simulink model "satellite2"  (R2025b)
settings: Solver=FixedStepAuto  StartTime=0.0  StopTime=5000  FixedStep=dt  MinStep=0.0001  RelTol=1e-3
values from neighbouring files (symbols this model uses):
  A_mw = [ ... (first row only)    [init_params.m]
  A_w = [ ... (first row only)    [init_params.m]
  alpha1 = 0.1    [init_params.m]
  alpha2 = 0.1    [init_params.m]
  angle0 = eAR'    [init_params.m]
  area_d = 4    [init_params.m]
  area_m2 = 0.0127    [init_params.m]
  area_s = 2    [init_params.m]
  ARW_deg_per_sqrt_h = 0.01    [init_params.m]
  B_mw = [ ... (first row only)    [init_params.m]
  beta1 = 0.01    [init_params.m]
  beta2 = 0.01    [init_params.m]
  bias0_deg_h = 0.01    [init_params.m]
  C_bus = 0.001    [init_params.m]
  C_mw = [ ... (first row only)    [init_params.m]
  Cd = 2.2    [init_params.m]
  cos_g_max = cos(gamma_max)    [init_params.m]
  Cr = 1.2    [init_params.m]
  D_max = 1    [init_params.m]
  Delta_D = 0.001    [init_params.m]
  dP_th = 0.05    [init_params.m]
  epsilon = 0.01    [init_params.m]
  eta = 0.7    [init_params.m]
  eta_buck = 0.9    [init_params.m]
  eta_chg = 0.95    [init_params.m]
  f = 2.2e9    (= 2200000000)    [init_params.m]
  f_n_hz = 400    [init_params.m]
  g0 = 9.80665    [init_params.m]
  G0 = 1366.1    [init_params.m]
  Gr_dB = 20    [init_params.m]
  Gt_dB = 3    [init_params.m]
  H = 50e3    (= 50000)    [init_params.m]
  h_ref = 400e3    (= 400000)    [init_params.m]
  hat_s = [1;0;0]    [init_params.m]
  I_chg_max = 8    [init_params.m]
  I_dis_max = 10    [init_params.m]
  I_e = 11    [init_params.m]
  I_gate = 0.5    [init_params.m]
  I_triggle = 8    [init_params.m]
  initial_phase = 0    [init_params.m]
  Isp = 220    [init_params.m]
  Iw = 0.02    [init_params.m]
  J2 = 1.08262668e-3    (= 0.00108262668)    [init_params.m]
  Jx = 10    [init_params.m]
  Jy = 12    [init_params.m]
  Jz = 8    [init_params.m]
  k_a = 4e-4    (= 0.0004)    [init_params.m]
  k_bias1_deg_h_per_C = 1    [init_params.m]
  k_bias2_deg_h_per_C = 0.0    (= 0)    [init_params.m]
  k_sf1_ppm = 1.0    (= 1)    [init_params.m]
  k_sf2_ppm = 0.0    (= 0)    [init_params.m]
  K_w = A_w' / (A_w * A_w')    [init_params.m]
  Kd = [ ... (first row only)    [init_params.m]
  kI = 0.01    [init_params.m]
  Kp = [ ... (first row only)    [init_params.m]
  kP = 10    [init_params.m]
  m = 500    [init_params.m]
  m0 = 20    [init_params.m]
  mu = 3.986004418e14    (= 398600441800000)    [init_params.m]
  n_solar = [1;0;0]    [init_params.m]
  omegaE = 7.2921159e-5    (= 7.2921159e-05)    [init_params.m]
  P0 = 4.56e-6    (= 4.56e-06)    [init_params.m]
  P_adcs = 20    [init_params.m]
  P_base = 50    [init_params.m]
  P_cc = 220/V_bus0    (= 7.85714285714)    [init_params.m]
  P_comm = 40    [init_params.m]
  P_prop = 5    [init_params.m]
  P_trickle = 14/V_bus0    (= 0.5)    [init_params.m]
  perimeter_m = 0.4    [init_params.m]
  Pt_dBW = 10    [init_params.m]
  Q = 20    [init_params.m]
  Q0 = [0.6;0.8;0;0]    [init_params.m]
  r1 = 1e-4    (= 0.0001)    [init_params.m]
  r2 = 1e-4    (= 0.0001)    [init_params.m]
  r_ref = 7.026e6    (= 7026000)    [init_params.m]
  Rb = 0.2    [init_params.m]
  Re = 6378137    [init_params.m]
  rho_ref = 3e-12    [init_params.m]
  rpm_max = 6000    [init_params.m]
  sf_factor = 0.85    [init_params.m]
  sigma1 = 0    [init_params.m]
  sigma2 = 0    [init_params.m]
  SOC0 = 0.6    [init_params.m]
  SOC1 = 0.2    [init_params.m]
  SOC2 = 0.8    [init_params.m]
  SOC_low_adcs = 0.1    [init_params.m]
  SOC_low_comm = 0.2    [init_params.m]
  SOC_low_prop = 0.2    [init_params.m]
  sta_vec = Re * [ ... (first row only)    [init_params.m]
  t_a = 0.1    [init_params.m]
  T_max = 0.05    [init_params.m]
  T_nominal = 20    [init_params.m]
  tau12 = 0.001    [init_params.m]
  tau21 = 0.001    [init_params.m]
  tau_th_s = 200    [init_params.m]
  tau_thr = 0.2    [init_params.m]
  theta12 = 0.005    [init_params.m]
  theta21 = 0.005    [init_params.m]
  V_bus0 = 28    [init_params.m]
  V_center = 50    [init_params.m]
  V_max = 33    [init_params.m]
  V_min = 24    [init_params.m]
  V_oc = num_s*Vmp    [init_params.m]
  v_peak_deg_s = 1.0    (= 1)    [init_params.m]
  V_pzt_max = 100    [init_params.m]
  V_pzt_min = 0    [init_params.m]
  vx0 = 0    [init_params.m]
  vy0 = 7546    [init_params.m]
  vz0 = 0    [init_params.m]
  w0 = [0;0;0]    [init_params.m]
  wavelength_m = 632.8e-9    (= 6.328e-07)    [init_params.m]
  white_rate_std_deg_s = 0    [init_params.m]
  x0 = 7e6    (= 7000000)    [init_params.m]
  y0 = 0    [init_params.m]
  z0 = 0    [init_params.m]
  zeta = 0.01    [init_params.m]
libraries: matrix_library x14, simulink x7, nesl_utility x4, simulink_extras x3, fl_lib x3, ee_lib x1
(part 2 of 2)

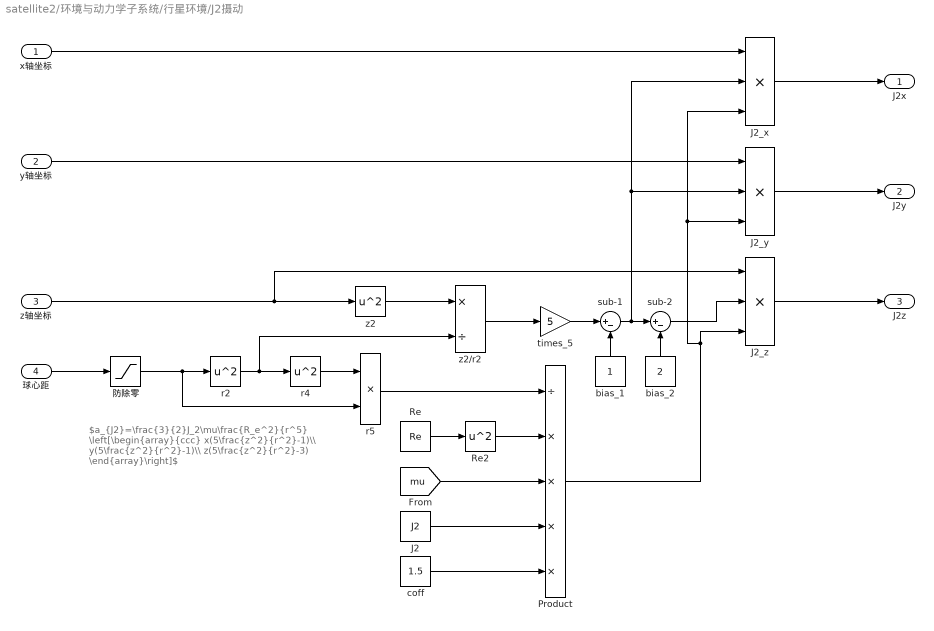
== system satellite2/环境与动力学子系统/行星环境/J2摄动 ==
  note: $a_{J2}=\frac{3}{2}J_2\mu\frac{R_e^2}{r^5} \left[\begin{array}{ccc} x(5\frac{z^2}{r^2}-1)\\ y(5\frac{z^2}{r^2}-1)\\ z(5\frac{z^2}{r^2}-3) \end{array}\right]$
  x轴坐标 : Inport
  y轴坐标 : Inport  Port=2
  z轴坐标 : Inport  Port=3
  球心距 : Inport  Port=4
  J2 : Constant  Value=J2
  J2_x : Product  Inputs=3
  J2_y : Product  Inputs=3
  J2_z : Product  Inputs=3
  Product : Product  Inputs=/****
  Re : Constant  Value=Re
  Re2 : Math  Operator=square
  bias_1 : Constant
  bias_2 : Constant  Value=2
  coff : Constant  Value=1.5
  r2 : Math  Operator=square
  r4 : Math  Operator=square
  r5 : Product
  sub-1 : Sum  Inputs=|+-
  sub-2 : Sum  Inputs=|+-
  times_5 : Gain  Gain=5
  z2 : Math  Operator=square
  z2/r2 : Product  Inputs=*/
  防除零 : Saturate  UpperLimit=inf  LowerLimit=Re+80e3
  J2x : Outport
  J2y : Outport  Port=2
  J2z : Outport  Port=3
  wires:
  Re2/1 -> Product/2
  z2/1 -> z2/r2/1
  x轴坐标/1 -> J2_x/1
  z2/r2/1 -> times_5/1
  sub-1/1 -> J2_y/2, J2_x/2, sub-2/1
  Product/1 -> J2_x/3, J2_y/3, J2_z/3
  coff/1 -> Product/5
  J2_z/1 -> J2z/1
  r4/1 -> r5/1
  z轴坐标/1 -> J2_z/1, z2/1
  r2/1 -> z2/r2/2, r4/1
  球心距/1 -> 防除零/1
  bias_1/1 -> sub-1/2
  [mu] -> Product/3
  times_5/1 -> sub-1/1
  sub-2/1 -> J2_z/2
  Re/1 -> Re2/1
  y轴坐标/1 -> J2_y/1
  J2/1 -> Product/4
  r5/1 -> Product/1
  bias_2/1 -> sub-2/2
  J2_y/1 -> J2y/1
  J2_x/1 -> J2x/1
  防除零/1 -> r5/2, r2/1

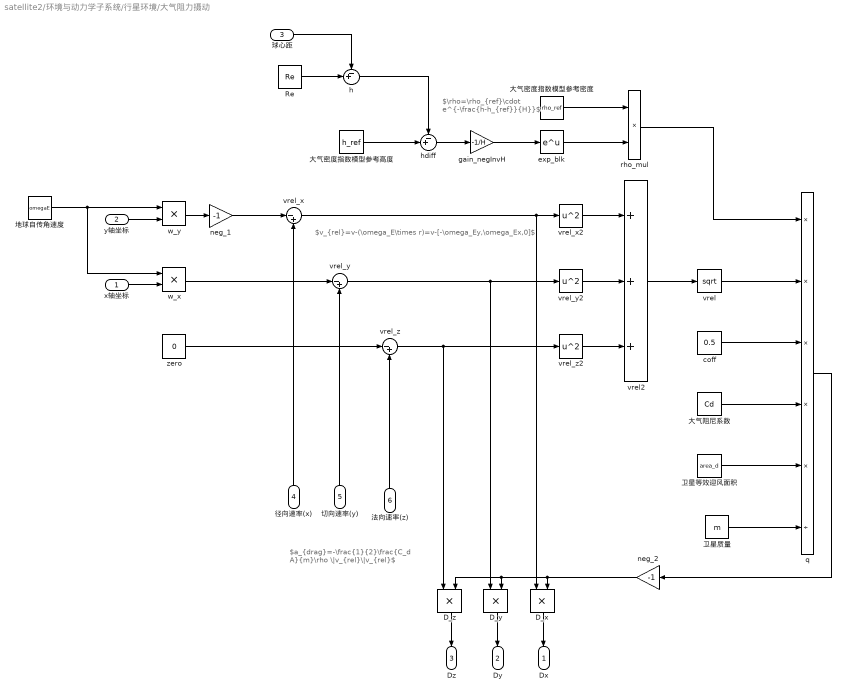
== system satellite2/环境与动力学子系统/行星环境/大气阻力摄动 ==
  note: $a_{drag}=-\frac{1}{2}\frac{C_d A}{m}\rho \|v_{rel}\|v_{rel}$
  note: $\rho=\rho_{ref}\cdot e^{-\frac{h-h_{ref}}{H}}$
  note: $v_{rel}=v-(\omega_E\times r)=v-[-\omega_Ey,\omega_Ex,0]$
  x轴坐标 : Inport
  y轴坐标 : Inport  Port=2
  球心距 : Inport  Port=3
  径向速率(x) : Inport  Port=4
  切向速率(y) : Inport  Port=5
  法向速率(z) : Inport  Port=6
  D_x : Product
  D_y : Product
  D_z : Product
  Re : Constant  Value=Re
  coff : Constant  Value=0.5
  exp_blk : Math
  gain_negInvH : Gain  Gain=-1/H
  h : Sum  Inputs=-+|
  hdiff : Sum  Inputs=-+|
  neg_1 : Gain  Gain=-1
  neg_2 : Gain  Gain=-1
  q : Product  Inputs=*****/
  rho_mul : Product
  vrel : Sqrt
  vrel2 : Sum  Inputs=+++
  vrel_x : Sum  Inputs=|-+
  vrel_x2 : Math  Operator=square
  vrel_y : Sum  Inputs=|-+
  vrel_y2 : Math  Operator=square
  vrel_z : Sum  Inputs=|-+
  vrel_z2 : Math  Operator=square
  w_x : Product
  w_y : Product
  zero : Constant  Value=0
  卫星等效迎风面积 : Constant  Value=area_d
  卫星质量 : Constant  Value=m
  地球自传角速度 : Constant  Value=omegaE
  大气密度指数模型参考密度 : Constant  Value=rho_ref
  大气密度指数模型参考高度 : Constant  Value=h_ref
  大气阻尼系数 : Constant  Value=Cd
  Dx : Outport
  Dy : Outport  Port=2
  Dz : Outport  Port=3
  wires:
  法向速率(z)/1 -> vrel_z/2
  切向速率(y)/1 -> vrel_y/2
  w_y/1 -> neg_1/1
  vrel_x/1 -> D_x/1, vrel_x2/1
  q/1 -> neg_2/1
  vrel_z2/1 -> vrel2/3
  vrel_x2/1 -> vrel2/1
  大气密度指数模型参考密度/1 -> rho_mul/1
  vrel2/1 -> vrel/1
  Re/1 -> h/2
  地球自传角速度/1 -> w_x/1, w_y/1
  x轴坐标/1 -> w_x/2
  neg_1/1 -> vrel_x/1
  vrel_y/1 -> D_y/1, vrel_y2/1
  D_z/1 -> Dz/1
  vrel_y2/1 -> vrel2/2
  coff/1 -> q/3
  rho_mul/1 -> q/1
  h/1 -> hdiff/1
  w_x/1 -> vrel_y/1
  卫星质量/1 -> q/6
  卫星等效迎风面积/1 -> q/5
  gain_negInvH/1 -> exp_blk/1
  zero/1 -> vrel_z/1
  径向速率(x)/1 -> vrel_x/2
  vrel_z/1 -> D_z/1, vrel_z2/1
  大气密度指数模型参考高度/1 -> hdiff/2
  hdiff/1 -> gain_negInvH/1
  vrel/1 -> q/2
  大气阻尼系数/1 -> q/4
  exp_blk/1 -> rho_mul/2
  y轴坐标/1 -> w_y/2
  球心距/1 -> h/1
  D_x/1 -> Dx/1
  D_y/1 -> Dy/1
  neg_2/1 -> D_x/2, D_y/2, D_z/2

== system satellite2/环境与动力学子系统/行星环境/太阳光压摄动 ==
  note: 后续对日矢量可完善
  三轴坐标 : Inport
  AND : Logic  AllPortsSameDT=off  OutDataTypeStr=boolean
  Add : Sum
  Demux : Demux  Outputs=3
  Demux1 : Demux  Outputs=3
  NOT : Logic  Operator=NOT  AllPortsSameDT=off  OutDataTypeStr=boolean
  Product : Product  Inputs=***/**
  Relational Operator : RelationalOperator  Operator=<  OutDataTypeStr=boolean  RndMeth=Simplest  InputSameDT=off
  Relational Operator1 : RelationalOperator  Operator=<  OutDataTypeStr=boolean  RndMeth=Simplest  InputSameDT=off
  Sqrt : Sqrt
  Square : Math  Operator=square
  Square1 : Math  Operator=square
  Zero : Constant  Value=0  OutDataTypeStr=Inherit: Inherit via back propagation
  卫星总质量 : Constant  Value=m
  受照面积 : Constant  Value=area_s
  地球半径 : Constant  Value=Re
  太阳辐射压强 : Constant  Value=P0
  对日单位方向矢量 : Constant  Value=hat_s
  辐射压系数 : Constant  Value=Cr
  srp_x : Outport
  srp_y : Outport  Port=2
  srp_z : Outport  Port=3
  wires:
  对日单位方向矢量/1 -> Product/5
  太阳辐射压强/1 -> Product/1
  卫星总质量/1 -> Product/4
  受照面积/1 -> Product/3
  辐射压系数/1 -> Product/2
  Product/1 -> Demux/1
  Demux/3 -> srp_z/1
  Demux/2 -> srp_y/1
  三轴坐标/1 -> Demux1/1
  Demux/1 -> srp_x/1
  Demux1/1 -> Relational Operator/1
  Zero/1 -> Relational Operator/2
  Demux1/2 -> Square/1
  Demux1/3 -> Square1/1
  Square/1 -> Add/1
  Square1/1 -> Add/2
  Add/1 -> Sqrt/1
  Sqrt/1 -> Relational Operator1/1
  地球半径/1 -> Relational Operator1/2
  Relational Operator1/1 -> AND/2
  Relational Operator/1 -> AND/1
  NOT/1 -> Product/6
  AND/1 -> NOT/1

== system satellite2/电源子系统/太阳能板/太阳板 ==
  q : Inport
  日照标志 : Inport  Port=2
  母线电压 : Inport  Port=3
  Max : MinMax  Function=max  Inputs=2
  eta : Gain  Gain=eta_buck
  伏电特性 : Subsystem
  入射角余弦 : Subsystem
  入射辐照度 : Switch  Criteria=u2 ~= 0  SaturateOnIntegerOverflow=off  InputSameDT=off
  最简单光生模型 : Gain  Gain=G0
  步进MPPT : Subsystem
  太阳板输出电流 : Outport
  wires:
  最简单光生模型/1 -> 入射辐照度/1  "I_ph"
  q/1 -> 入射角余弦/1(q)
  日照标志/1 -> 入射辐照度/2
  入射角余弦/1(入射角余弦) -> 最简单光生模型/1
  [zero] -> Max/2, 入射辐照度/3
  Max/1 -> eta/1, 步进MPPT/1(I_panel)  "I_panel"
  eta/1 -> 太阳板输出电流/1
  入射辐照度/1 -> 伏电特性/1(lr)
  伏电特性/1(I) -> Max/1
  母线电压/1 -> 步进MPPT/2(母线电压)
  步进MPPT/1(太阳电池电压) -> 伏电特性/2(V)

== system satellite2/电源子系统/视线角标志/余弦夹角 ==
  u1 : Inport
  u2 : Inport  Port=2
  Demux : Demux  Outputs=3
  Demux1 : Demux  Outputs=3
  Dot Product : DotProduct  OutDataTypeStr=Inherit: Inherit via internal rule
  余弦夹角 : Product  Inputs=/*/
  向量模长-r1 : Subsystem
  向量模长-r2 : Subsystem
  cos(γ) : Outport
  wires:
  向量模长-r2/1(|u|) -> 余弦夹角/3
  Demux/3 -> 向量模长-r1/3(u3)
  Demux/2 -> 向量模长-r1/2(u2)
  Dot Product/1 -> 余弦夹角/2
  Demux/1 -> 向量模长-r1/1(u1)
  向量模长-r1/1(|u|) -> 余弦夹角/1
  u2/1 -> Dot Product/2, Demux1/1
  Demux1/1 -> 向量模长-r2/1(u1)
  Demux1/2 -> 向量模长-r2/2(u2)
  Demux1/3 -> 向量模长-r2/3(u3)
  u1/1 -> Dot Product/1, Demux/1
  余弦夹角/1 -> cos(γ)/1

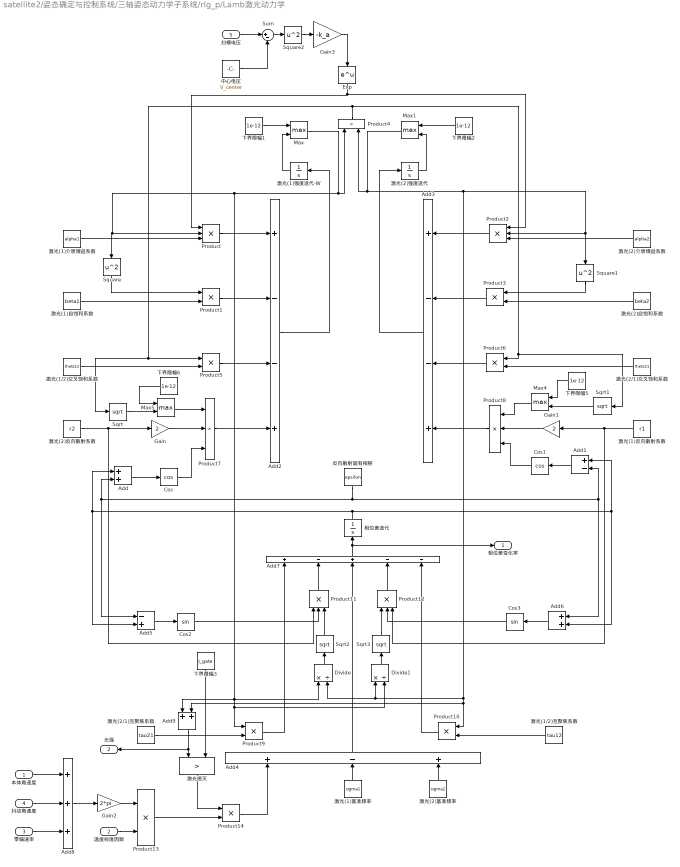
== system satellite2/姿态确定与控制系统/三轴姿态动力学子系统/rlg_p/Lamb激光动力学 ==
  本体角速度 : Inport
  温度标度因数 : Inport  Port=2
  零偏速率 : Inport  Port=3
  抖动角速度 : Inport  Port=4
  扫模电压 : Inport  Port=5
  Add : Sum
  Add1 : Sum  Inputs=+-
  Add2 : Sum  Inputs=+--+
  Add3 : Sum  Inputs=+--+
  Add4 : Sum  Inputs=+-+
  Add5 : Sum  Inputs=-+
  Add6 : Sum
  Add7 : Sum  Inputs=+-+--
  Add8 : Sum  Inputs=+++
  Add9 : Sum
  Cos : Trigonometry  Operator=cos
  Cos1 : Trigonometry  Operator=cos
  Cos2 : Trigonometry
  Cos3 : Trigonometry
  Divide : Product  Inputs=*/
  Divide1 : Product  Inputs=*/
  Exp : Math
  Gain : Gain  Gain=2
  Gain1 : Gain  Gain=2
  Gain2 : Gain  Gain=2*pi
  Gain3 : Gain  Gain=-k_a
  Max{,1,4..5} (4 alike) : MinMax  Function=max  Inputs=2
  Product{,2,7..8,11..12} (6 alike) : Product  Inputs=3
  Product{1,3..6,9..10,13..14} (9 alike) : Product
  Sqrt{,1..3} (4 alike) : Sqrt
  Square : Math  Operator=square
  Square1 : Math  Operator=square
  Square2 : Math  Operator=square
  Sum : Sum  Inputs=|+-
  下界限幅{1..2,5..6} (4 alike) : Constant  Value=1e-12
  下界限幅3 : Constant  Value=I_gate
  中心电压 : Constant  Value=V_center
  反向散射固有相移 : Constant  Value=epsilon
  激光(1)介质增益系数 : Constant  Value=alpha1
  激光(1)反向散射系数 : Constant  Value=r1
  激光(1)基准频率 : Constant  Value=sigma1
  激光(1)强度迭代-W : Integrator  InitialCondition=1
  激光(1)自饱和系数 : Constant  Value=beta1
  激光(1/2)互聚焦系数 : Constant  Value=tau12
  激光(1/2)交叉饱和系数 : Constant  Value=theta12
  激光(2)介质增益系数 : Constant  Value=alpha2
  激光(2)反向散射系数 : Constant  Value=r2
  激光(2)基准频率 : Constant  Value=sigma2
  激光(2)强度迭代 : Integrator  InitialCondition=1
  激光(2)自饱和系数 : Constant  Value=beta2
  激光(2/1)互聚焦系数 : Constant  Value=tau21
  激光(2/1)交叉饱和系数 : Constant  Value=theta21
  激光熄灭 : RelationalOperator  Operator=>  OutDataTypeStr=boolean  InputSameDT=off
  相位差迭代 : Integrator
  相位差变化率 : Outport
  光强 : Outport  Port=2
  wires:
  激光(1)介质增益系数/1 -> Product/3
  激光(1)自饱和系数/1 -> Product1/2
  Square/1 -> Product1/1
  激光(2)介质增益系数/1 -> Product2/3
  激光(2)自饱和系数/1 -> Product3/2
  Square1/1 -> Product3/1
  激光(1/2)交叉饱和系数/1 -> Product5/2
  激光(2/1)交叉饱和系数/1 -> Product6/2
  下界限幅1/1 -> Max/1
  Product4/1 -> Product6/1, Sqrt1/1, Product5/1, Sqrt/1
  激光(2)反向散射系数/1 -> Gain/1, Product11/1
  Gain/1 -> Product7/2
  Max5/1 -> Product7/1
  Cos/1 -> Product7/3
  Add/1 -> Cos/1
  反向散射固有相移/1 -> Add1/2, Add6/1, Add5/1, Add/2
  Cos1/1 -> Product8/3
  Max4/1 -> Product8/1
  Add1/1 -> Cos1/1
  Gain1/1 -> Product8/2
  激光(1)反向散射系数/1 -> Product12/3, Gain1/1
  下界限幅2/1 -> Max1/1
  Product/1 -> Add2/1
  Product1/1 -> Add2/2
  Product5/1 -> Add2/3
  Add2/1 -> 激光(1)强度迭代-W/1
  Product2/1 -> Add3/1
  Product3/1 -> Add3/2
  Product6/1 -> Add3/3
  Product8/1 -> Add3/4
  Add3/1 -> 激光(2)强度迭代/1
  激光(2/1)互聚焦系数/1 -> Product9/2
  激光(1/2)互聚焦系数/1 -> Product10/2
  Product7/1 -> Add2/4
  Add5/1 -> Cos2/1
  Max/1 -> Add9/1, Product9/1, Divide1/2, Divide/1, Product/2, Square/1, Product4/1
  Divide/1 -> Sqrt2/1
  Cos2/1 -> Product11/2
  相位差迭代/1 -> Add1/1, Add6/2, Add5/2, Add/1
  Add6/1 -> Cos3/1
  Divide1/1 -> Sqrt3/1
  Cos3/1 -> Product12/2
  激光(1)基准频率/1 -> Add4/2
  激光(2)基准频率/1 -> Add4/3
  Product14/1 -> Add4/1
  Product9/1 -> Add7/1
  Product10/1 -> Add7/5
  Product11/1 -> Add7/2
  Product12/1 -> Add7/4
  Add4/1 -> Add7/3
  Add7/1 -> 相位差变化率/1, 相位差迭代/1
  激光(1)强度迭代-W/1 -> Max/2
  激光(2)强度迭代/1 -> Max1/2
  下界限幅5/1 -> Max4/1
  Sqrt1/1 -> Max4/2
  下界限幅6/1 -> Max5/1
  Sqrt/1 -> Max5/2
  Sqrt2/1 -> Product11/3
  Sqrt3/1 -> Product12/1
  零偏速率/1 -> Add8/3
  温度标度因数/1 -> Product13/2
  本体角速度/1 -> Add8/1
  抖动角速度/1 -> Add8/2
  Add8/1 -> Gain2/1
  Gain2/1 -> Product13/1
  Max1/1 -> Product4/2, Square1/1, Product2/2, Divide/2, Divide1/1, Add9/2, Product10/1
  Add9/1 -> 光强/1, 激光熄灭/1
  Product13/1 -> Product14/2
  激光熄灭/1 -> Product14/1
  下界限幅3/1 -> 激光熄灭/2
  扫模电压/1 -> Sum/1
  中心电压/1 -> Sum/2
  Sum/1 -> Square2/1
  Gain3/1 -> Exp/1
  Exp/1 -> Product2/1, Product/1
  Square2/1 -> Gain3/1

== system satellite2/姿态确定与控制系统/三轴姿态动力学子系统/rlg_p/几何参数 ==
  Mux : Mux  Inputs=3
  激光波长-m : Constant  Value=wavelength_m
  环形腔周长-m : Constant  Value=perimeter_m
  环形腔面积-m2 : Constant  Value=area_m2
  计算集合标度因数-S0 : Fcn  Expr=4*u(1)/(u(2)*u(3))
  标度因数 : Outport
  wires:
  计算集合标度因数-S0/1 -> 标度因数/1
  Mux/1 -> 计算集合标度因数-S0/1
  环形腔面积-m2/1 -> Mux/1
  激光波长-m/1 -> Mux/2
  环形腔周长-m/1 -> Mux/3

== system satellite2/姿态确定与控制系统/三轴姿态动力学子系统/rlg_p/噪声模型 ==
  标度因数 : Inport
  相位差变化率 : Inport  Port=2
  Add : Sum
  Band-Limited White Noise : simulink/Sources/Band-Limited White Noise  Cov=[(ARW_deg_per_sqrt_h/60)^2 + white_rate_std_deg_s^2]  Ts=1  seed=[23341]
  Divide : Product  Inputs=/*
  Gain : Gain  Gain=pi/180
  r2Hz : Gain  Gain=1/(2*pi)
  测量角速度 : Outport
  wires:
  Add/1 -> 测量角速度/1
  r2Hz/1 -> Divide/2
  Gain/1 -> Add/1
  Band-Limited White Noise/1 -> Gain/1
  Divide/1 -> Add/2
  相位差变化率/1 -> r2Hz/1
  标度因数/1 -> Divide/1

== system satellite2/姿态确定与控制系统/三轴姿态动力学子系统/rlg_p/控模与扫模逻辑 ==
  光强 : Inport
  Add : Sum  Inputs=+-
  Add1 : Sum
  Gain : Gain  Gain=kP
  Gain1 : Gain  Gain=kI
  Integrator : Integrator
  Switch : Switch  Criteria=u2 > Threshold  SaturateOnIntegerOverflow=off  InputSameDT=off
  zero : Constant  Value=0  OutDataTypeStr=boolean
  光强阈值 : Constant  Value=I_triggle
  扫模信号发生器 : simulink/Sources/Repeating Sequence  rep_seq_t=[0 0.5 1]  rep_seq_y=[0 V_pzt_max V_pzt_min]
  期望光强 : Constant  Value=I_e
  状态切换 : simulink_extras/Flip Flops/S-R Flip-Flop  initial_condition=0
  触发信号 : RelationalOperator  OutDataTypeStr=boolean  RndMeth=Simplest  InputSameDT=off
  触发信号1 : RelationalOperator  Operator=<  OutDataTypeStr=boolean  RndMeth=Simplest  InputSameDT=off
  跌落阈值 : Constant  Value=I_gate
  扫模电压 : Outport
  wires:
  光强阈值/1 -> 触发信号/2
  期望光强/1 -> Add/1
  Add1/1 -> Switch/1
  状态切换/1 -> Switch/2
  扫模信号发生器/1 -> Switch/3
  触发信号/1 -> 状态切换/1
  Switch/1 -> 扫模电压/1
  Add/1 -> Gain1/1, Gain/1
  Gain/1 -> Add1/2
  Gain1/1 -> Integrator/1
  Integrator/1 -> Add1/1
  触发信号1/1 -> 状态切换/2
  光强/1 -> 触发信号1/1, Add/2, 触发信号/1
  跌落阈值/1 -> 触发信号1/2

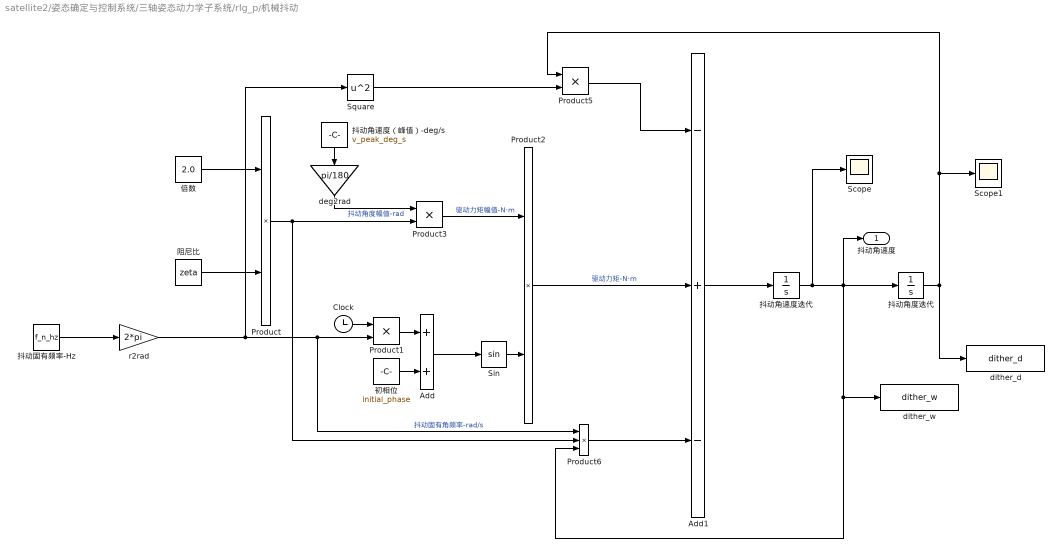
== system satellite2/姿态确定与控制系统/三轴姿态动力学子系统/rlg_p/机械抖动 ==
  Add : Sum
  Add1 : Sum  Inputs=-+-
  Clock : Clock
  Product{,1..3,5} (5 alike) : Product
  Product6 : Product  Inputs=3
  Scope : Scope
      settings: DataLoggingVariableName=ScopeData4
  Scope1 : Scope
      settings: DataLoggingVariableName=ScopeData5
  Sin : Trigonometry
  Square : Math  Operator=square
  deg2rad : Gain  Gain=pi/180
  dither_d : ToWorkspace  VariableName=dither_d  SampleTime=-1
  dither_w : ToWorkspace  VariableName=dither_w  SampleTime=-1
  r2rad : Gain  Gain=2*pi
  倍数 : Constant  Value=2.0
  初相位 : Constant  Value=initial_phase
  抖动固有频率-Hz : Constant  Value=f_n_hz
  抖动角度迭代 : Integrator
  抖动角速度迭代 : Integrator
  抖动角速度（峰值）-deg/s : Constant  Value=v_peak_deg_s
  阻尼比 : Constant  Value=zeta
  抖动角速度 : Outport
  wires:
  r2rad/1 -> Square/1, Product6/1, Product1/2  "抖动固有角频率-rad/s"
  抖动固有频率-Hz/1 -> r2rad/1
  阻尼比/1 -> Product/2
  倍数/1 -> Product/1
  Clock/1 -> Product1/1
  Product1/1 -> Add/1
  初相位/1 -> Add/2
  Add/1 -> Sin/1
  Product3/1 -> Product2/1  "驱动力矩幅值-N·m"
  Sin/1 -> Product2/2
  Product2/1 -> Add1/2  "驱动力矩-N·m"
  deg2rad/1 -> Product3/1  "抖动角度幅值-rad"
  抖动角速度（峰值）-deg/s/1 -> deg2rad/1
  Product/1 -> Product6/2, Product3/2
  Add1/1 -> 抖动角速度迭代/1
  Product6/1 -> Add1/3
  Square/1 -> Product5/2
  抖动角度迭代/1 -> dither_d/1, Scope1/1, Product5/1
  Product5/1 -> Add1/1
  抖动角速度迭代/1 -> Scope/1, dither_w/1, Product6/3, 抖动角速度/1, 抖动角度迭代/1

== system satellite2/姿态确定与控制系统/三轴姿态动力学子系统/rlg_p/热模型 ==
  环境温度-°C : Inport
  几何标度因数 : Inport  Port=2
  Add : Sum
  Add1 : Sum  Inputs=+++
  Add2 : Sum
  Product : Product
  Sum : Sum  Inputs=|-+
  deg2rad(s) : Gain  Gain=pi/(180*3600)
  平方 : Math  Operator=square
  标定/初始温度 : Constant  Value=25
  标度因数倍数（参考温度） : Constant
  比较 : Sum  Inputs=-+|
  温度标度因数系数（1阶） : Gain  Gain=k_sf1_ppm
  温度标度因数系数（2阶） : Gain  Gain=k_sf2_ppm
  温度迭代 : Integrator  InitialConditionSource=external  InitialCondition=25.0
  温度零偏系数（1阶） : Gain  Gain=k_bias1_deg_h_per_C
  温度零偏系数（2阶） : Gain  Gain=k_bias2_deg_h_per_C
  热时间常数 : Gain  Gain=1/tau_th_s
  百万分之一每摄氏度 : Gain  Gain=1e-6
  零偏（参考温度） : Constant  Value=bias0_deg_h
  陀螺温度-°C : Outport
  温度标度因数 : Outport  Port=2
  温度零偏 : Outport  Port=3
  wires:
  热时间常数/1 -> 温度迭代/1
  温度迭代/1 -> 陀螺温度-°C/1, Sum/2, 比较/1
  环境温度-°C/1 -> 比较/2
  比较/1 -> 热时间常数/1
  温度标度因数系数（1阶）/1 -> Add/1
  温度标度因数系数（2阶）/1 -> Add/2
  标定/初始温度/1 -> Sum/1, 温度迭代/2
  Add/1 -> 百万分之一每摄氏度/1
  Product/1 -> 温度标度因数/1
  平方/1 -> 温度标度因数系数（2阶）/1, 温度零偏系数（2阶）/1
  deg2rad(s)/1 -> 温度零偏/1
  几何标度因数/1 -> Product/1
  Add1/1 -> deg2rad(s)/1
  Sum/1 -> 平方/1, 温度标度因数系数（1阶）/1, 温度零偏系数（1阶）/1
  温度零偏系数（2阶）/1 -> Add1/3
  温度零偏系数（1阶）/1 -> Add1/2
  零偏（参考温度）/1 -> Add1/1
  百万分之一每摄氏度/1 -> Add2/2
  标度因数倍数（参考温度）/1 -> Add2/1
  Add2/1 -> Product/2

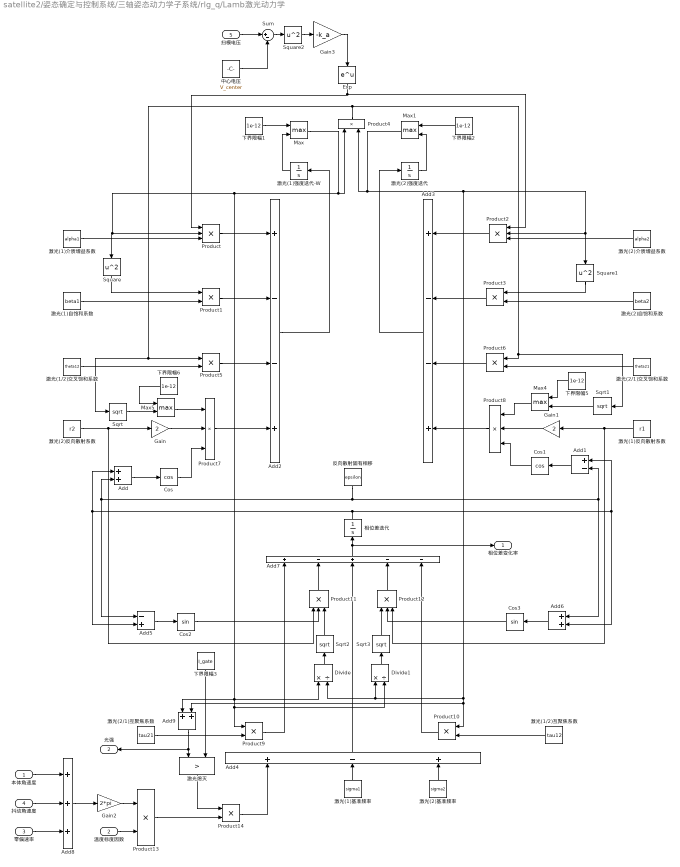
== system satellite2/姿态确定与控制系统/三轴姿态动力学子系统/rlg_q/Lamb激光动力学 ==
  本体角速度 : Inport
  温度标度因数 : Inport  Port=2
  零偏速率 : Inport  Port=3
  抖动角速度 : Inport  Port=4
  扫模电压 : Inport  Port=5
  Add : Sum
  Add1 : Sum  Inputs=+-
  Add2 : Sum  Inputs=+--+
  Add3 : Sum  Inputs=+--+
  Add4 : Sum  Inputs=+-+
  Add5 : Sum  Inputs=-+
  Add6 : Sum
  Add7 : Sum  Inputs=+-+--
  Add8 : Sum  Inputs=+++
  Add9 : Sum
  Cos : Trigonometry  Operator=cos
  Cos1 : Trigonometry  Operator=cos
  Cos2 : Trigonometry
  Cos3 : Trigonometry
  Divide : Product  Inputs=*/
  Divide1 : Product  Inputs=*/
  Exp : Math
  Gain : Gain  Gain=2
  Gain1 : Gain  Gain=2
  Gain2 : Gain  Gain=2*pi
  Gain3 : Gain  Gain=-k_a
  Max{,1,4..5} (4 alike) : MinMax  Function=max  Inputs=2
  Product{,2,7..8,11..12} (6 alike) : Product  Inputs=3
  Product{1,3..6,9..10,13..14} (9 alike) : Product
  Sqrt{,1..3} (4 alike) : Sqrt
  Square : Math  Operator=square
  Square1 : Math  Operator=square
  Square2 : Math  Operator=square
  Sum : Sum  Inputs=|+-
  下界限幅{1..2,5..6} (4 alike) : Constant  Value=1e-12
  下界限幅3 : Constant  Value=I_gate
  中心电压 : Constant  Value=V_center
  反向散射固有相移 : Constant  Value=epsilon
  激光(1)介质增益系数 : Constant  Value=alpha1
  激光(1)反向散射系数 : Constant  Value=r1
  激光(1)基准频率 : Constant  Value=sigma1
  激光(1)强度迭代-W : Integrator  InitialCondition=1
  激光(1)自饱和系数 : Constant  Value=beta1
  激光(1/2)互聚焦系数 : Constant  Value=tau12
  激光(1/2)交叉饱和系数 : Constant  Value=theta12
  激光(2)介质增益系数 : Constant  Value=alpha2
  激光(2)反向散射系数 : Constant  Value=r2
  激光(2)基准频率 : Constant  Value=sigma2
  激光(2)强度迭代 : Integrator  InitialCondition=1
  激光(2)自饱和系数 : Constant  Value=beta2
  激光(2/1)互聚焦系数 : Constant  Value=tau21
  激光(2/1)交叉饱和系数 : Constant  Value=theta21
  激光熄灭 : RelationalOperator  Operator=>  OutDataTypeStr=boolean  InputSameDT=off
  相位差迭代 : Integrator
  相位差变化率 : Outport
  光强 : Outport  Port=2
  wires:
  Square2/1 -> Gain3/1
  Exp/1 -> Product/1, Product2/1
  Gain3/1 -> Exp/1
  Sum/1 -> Square2/1
  中心电压/1 -> Sum/2
  扫模电压/1 -> Sum/1
  下界限幅3/1 -> 激光熄灭/2
  激光熄灭/1 -> Product14/1
  Product13/1 -> Product14/2
  Add9/1 -> 激光熄灭/1, 光强/1
  Max1/1 -> Product10/1, Add9/2, Divide1/1, Divide/2, Product2/2, Square1/1, Product4/2
  Gain2/1 -> Product13/1
  Add8/1 -> Gain2/1
  抖动角速度/1 -> Add8/2
  本体角速度/1 -> Add8/1
  温度标度因数/1 -> Product13/2
  零偏速率/1 -> Add8/3
  Sqrt3/1 -> Product12/1
  Sqrt2/1 -> Product11/3
  Sqrt/1 -> Max5/2
  下界限幅6/1 -> Max5/1
  Sqrt1/1 -> Max4/2
  下界限幅5/1 -> Max4/1
  激光(2)强度迭代/1 -> Max1/2
  激光(1)强度迭代-W/1 -> Max/2
  Add7/1 -> 相位差迭代/1, 相位差变化率/1
  Add4/1 -> Add7/3
  Product12/1 -> Add7/4
  Product11/1 -> Add7/2
  Product10/1 -> Add7/5
  Product9/1 -> Add7/1
  Product14/1 -> Add4/1
  激光(2)基准频率/1 -> Add4/3
  激光(1)基准频率/1 -> Add4/2
  Cos3/1 -> Product12/2
  Divide1/1 -> Sqrt3/1
  Add6/1 -> Cos3/1
  相位差迭代/1 -> Add/1, Add5/2, Add6/2, Add1/1
  Cos2/1 -> Product11/2
  Divide/1 -> Sqrt2/1
  Max/1 -> Product4/1, Square/1, Product/2, Divide/1, Divide1/2, Product9/1, Add9/1
  Add5/1 -> Cos2/1
  Product7/1 -> Add2/4
  激光(1/2)互聚焦系数/1 -> Product10/2
  激光(2/1)互聚焦系数/1 -> Product9/2
  Add3/1 -> 激光(2)强度迭代/1
  Product8/1 -> Add3/4
  Product6/1 -> Add3/3
  Product3/1 -> Add3/2
  Product2/1 -> Add3/1
  Add2/1 -> 激光(1)强度迭代-W/1
  Product5/1 -> Add2/3
  Product1/1 -> Add2/2
  Product/1 -> Add2/1
  下界限幅2/1 -> Max1/1
  激光(1)反向散射系数/1 -> Gain1/1, Product12/3
  Gain1/1 -> Product8/2
  Add1/1 -> Cos1/1
  Max4/1 -> Product8/1
  Cos1/1 -> Product8/3
  反向散射固有相移/1 -> Add/2, Add5/1, Add6/1, Add1/2
  Add/1 -> Cos/1
  Cos/1 -> Product7/3
  Max5/1 -> Product7/1
  Gain/1 -> Product7/2
  激光(2)反向散射系数/1 -> Product11/1, Gain/1
  Product4/1 -> Sqrt/1, Product5/1, Sqrt1/1, Product6/1
  下界限幅1/1 -> Max/1
  激光(2/1)交叉饱和系数/1 -> Product6/2
  激光(1/2)交叉饱和系数/1 -> Product5/2
  Square1/1 -> Product3/1
  激光(2)自饱和系数/1 -> Product3/2
  激光(2)介质增益系数/1 -> Product2/3
  Square/1 -> Product1/1
  激光(1)自饱和系数/1 -> Product1/2
  激光(1)介质增益系数/1 -> Product/3

== system satellite2/姿态确定与控制系统/三轴姿态动力学子系统/rlg_q/几何参数 ==
  Mux : Mux  Inputs=3
  激光波长-m : Constant  Value=wavelength_m
  环形腔周长-m : Constant  Value=perimeter_m
  环形腔面积-m2 : Constant  Value=area_m2
  计算集合标度因数-S0 : Fcn  Expr=4*u(1)/(u(2)*u(3))
  标度因数 : Outport
  wires:
  环形腔周长-m/1 -> Mux/3
  激光波长-m/1 -> Mux/2
  环形腔面积-m2/1 -> Mux/1
  Mux/1 -> 计算集合标度因数-S0/1
  计算集合标度因数-S0/1 -> 标度因数/1

== system satellite2/姿态确定与控制系统/三轴姿态动力学子系统/rlg_q/噪声模型 ==
  标度因数 : Inport
  相位差变化率 : Inport  Port=2
  Add : Sum
  Band-Limited White Noise : simulink/Sources/Band-Limited White Noise  Cov=[(ARW_deg_per_sqrt_h/60)^2 + white_rate_std_deg_s^2]  Ts=1  seed=[23341]
  Divide : Product  Inputs=/*
  Gain : Gain  Gain=pi/180
  r2Hz : Gain  Gain=1/(2*pi)
  测量角速度 : Outport
  wires:
  标度因数/1 -> Divide/1
  相位差变化率/1 -> r2Hz/1
  Divide/1 -> Add/2
  Band-Limited White Noise/1 -> Gain/1
  Gain/1 -> Add/1
  r2Hz/1 -> Divide/2
  Add/1 -> 测量角速度/1

== system satellite2/姿态确定与控制系统/三轴姿态动力学子系统/rlg_q/控模与扫模逻辑 ==
  光强 : Inport
  Add : Sum  Inputs=+-
  Add1 : Sum
  Gain : Gain  Gain=kP
  Gain1 : Gain  Gain=kI
  Integrator : Integrator
  Switch : Switch  Criteria=u2 > Threshold  SaturateOnIntegerOverflow=off  InputSameDT=off
  zero : Constant  Value=0  OutDataTypeStr=boolean
  光强阈值 : Constant  Value=I_triggle
  扫模信号发生器 : simulink/Sources/Repeating Sequence  rep_seq_t=[0 0.5 1]  rep_seq_y=[0 V_pzt_max V_pzt_min]
  期望光强 : Constant  Value=I_e
  状态切换 : simulink_extras/Flip Flops/S-R Flip-Flop  initial_condition=0
  触发信号 : RelationalOperator  OutDataTypeStr=boolean  RndMeth=Simplest  InputSameDT=off
  触发信号1 : RelationalOperator  Operator=<  OutDataTypeStr=boolean  RndMeth=Simplest  InputSameDT=off
  跌落阈值 : Constant  Value=I_gate
  扫模电压 : Outport
  wires:
  跌落阈值/1 -> 触发信号1/2
  光强/1 -> 触发信号/1, Add/2, 触发信号1/1
  触发信号1/1 -> 状态切换/2
  Integrator/1 -> Add1/1
  Gain1/1 -> Integrator/1
  Gain/1 -> Add1/2
  Add/1 -> Gain/1, Gain1/1
  Switch/1 -> 扫模电压/1
  触发信号/1 -> 状态切换/1
  扫模信号发生器/1 -> Switch/3
  状态切换/1 -> Switch/2
  Add1/1 -> Switch/1
  期望光强/1 -> Add/1
  光强阈值/1 -> 触发信号/2

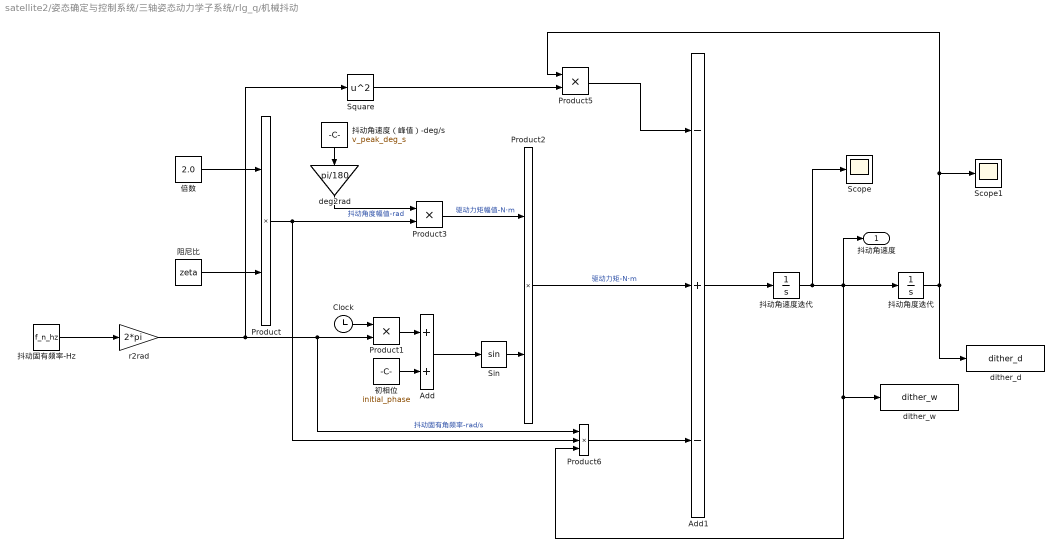
== system satellite2/姿态确定与控制系统/三轴姿态动力学子系统/rlg_q/机械抖动 ==
  Add : Sum
  Add1 : Sum  Inputs=-+-
  Clock : Clock
  Product{,1..3,5} (5 alike) : Product
  Product6 : Product  Inputs=3
  Scope : Scope
      settings: DataLoggingVariableName=ScopeData4
  Scope1 : Scope
      settings: DataLoggingVariableName=ScopeData5
  Sin : Trigonometry
  Square : Math  Operator=square
  deg2rad : Gain  Gain=pi/180
  dither_d : ToWorkspace  VariableName=dither_d  SampleTime=-1
  dither_w : ToWorkspace  VariableName=dither_w  SampleTime=-1
  r2rad : Gain  Gain=2*pi
  倍数 : Constant  Value=2.0
  初相位 : Constant  Value=initial_phase
  抖动固有频率-Hz : Constant  Value=f_n_hz
  抖动角度迭代 : Integrator
  抖动角速度迭代 : Integrator
  抖动角速度（峰值）-deg/s : Constant  Value=v_peak_deg_s
  阻尼比 : Constant  Value=zeta
  抖动角速度 : Outport
  wires:
  抖动角速度迭代/1 -> 抖动角度迭代/1, 抖动角速度/1, Product6/3, dither_w/1, Scope/1
  Product5/1 -> Add1/1
  抖动角度迭代/1 -> Product5/1, Scope1/1, dither_d/1
  Square/1 -> Product5/2
  Product6/1 -> Add1/3
  Add1/1 -> 抖动角速度迭代/1
  Product/1 -> Product3/2, Product6/2
  抖动角速度（峰值）-deg/s/1 -> deg2rad/1
  deg2rad/1 -> Product3/1  "抖动角度幅值-rad"
  Product2/1 -> Add1/2  "驱动力矩-N·m"
  Sin/1 -> Product2/2
  Product3/1 -> Product2/1  "驱动力矩幅值-N·m"
  Add/1 -> Sin/1
  初相位/1 -> Add/2
  Product1/1 -> Add/1
  Clock/1 -> Product1/1
  倍数/1 -> Product/1
  阻尼比/1 -> Product/2
  抖动固有频率-Hz/1 -> r2rad/1
  r2rad/1 -> Product1/2, Product6/1, Square/1  "抖动固有角频率-rad/s"

== system satellite2/姿态确定与控制系统/三轴姿态动力学子系统/rlg_q/热模型 ==
  环境温度-°C : Inport
  几何标度因数 : Inport  Port=2
  Add : Sum
  Add1 : Sum  Inputs=+++
  Add2 : Sum
  Product : Product
  Sum : Sum  Inputs=|-+
  deg2rad(s) : Gain  Gain=pi/(180*3600)
  平方 : Math  Operator=square
  标定/初始温度 : Constant  Value=25
  标度因数倍数（参考温度） : Constant
  比较 : Sum  Inputs=-+|
  温度标度因数系数（1阶） : Gain  Gain=k_sf1_ppm
  温度标度因数系数（2阶） : Gain  Gain=k_sf2_ppm
  温度迭代 : Integrator  InitialConditionSource=external  InitialCondition=25.0
  温度零偏系数（1阶） : Gain  Gain=k_bias1_deg_h_per_C
  温度零偏系数（2阶） : Gain  Gain=k_bias2_deg_h_per_C
  热时间常数 : Gain  Gain=1/tau_th_s
  百万分之一每摄氏度 : Gain  Gain=1e-6
  零偏（参考温度） : Constant  Value=bias0_deg_h
  陀螺温度-°C : Outport
  温度标度因数 : Outport  Port=2
  温度零偏 : Outport  Port=3
  wires:
  Add2/1 -> Product/2
  标度因数倍数（参考温度）/1 -> Add2/1
  百万分之一每摄氏度/1 -> Add2/2
  零偏（参考温度）/1 -> Add1/1
  温度零偏系数（1阶）/1 -> Add1/2
  温度零偏系数（2阶）/1 -> Add1/3
  Sum/1 -> 温度零偏系数（1阶）/1, 温度标度因数系数（1阶）/1, 平方/1
  Add1/1 -> deg2rad(s)/1
  几何标度因数/1 -> Product/1
  deg2rad(s)/1 -> 温度零偏/1
  平方/1 -> 温度零偏系数（2阶）/1, 温度标度因数系数（2阶）/1
  Product/1 -> 温度标度因数/1
  Add/1 -> 百万分之一每摄氏度/1
  标定/初始温度/1 -> 温度迭代/2, Sum/1
  温度标度因数系数（2阶）/1 -> Add/2
  温度标度因数系数（1阶）/1 -> Add/1
  比较/1 -> 热时间常数/1
  环境温度-°C/1 -> 比较/2
  温度迭代/1 -> 比较/1, Sum/2, 陀螺温度-°C/1
  热时间常数/1 -> 温度迭代/1

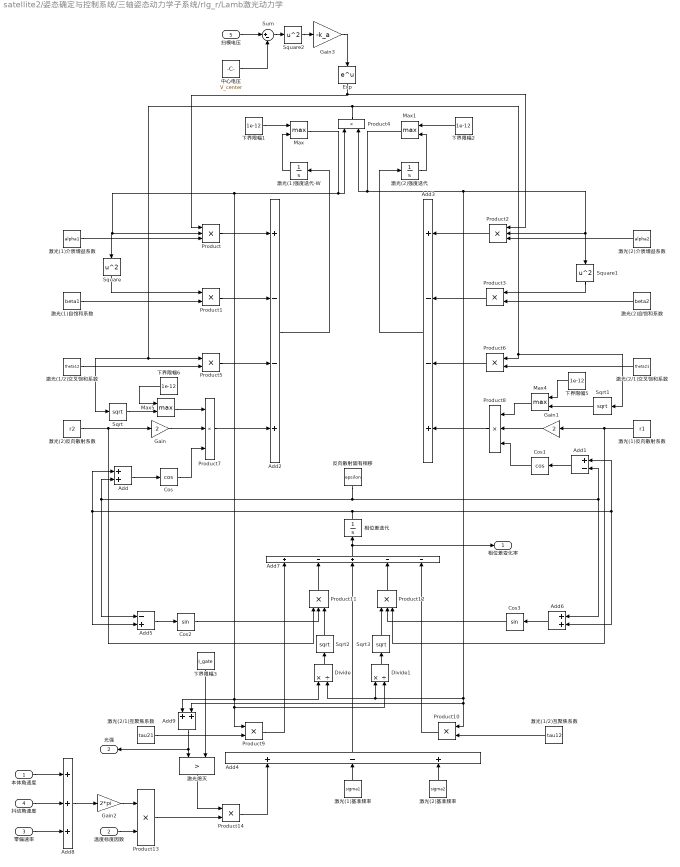
== system satellite2/姿态确定与控制系统/三轴姿态动力学子系统/rlg_r/Lamb激光动力学 ==
  本体角速度 : Inport
  温度标度因数 : Inport  Port=2
  零偏速率 : Inport  Port=3
  抖动角速度 : Inport  Port=4
  扫模电压 : Inport  Port=5
  Add : Sum
  Add1 : Sum  Inputs=+-
  Add2 : Sum  Inputs=+--+
  Add3 : Sum  Inputs=+--+
  Add4 : Sum  Inputs=+-+
  Add5 : Sum  Inputs=-+
  Add6 : Sum
  Add7 : Sum  Inputs=+-+--
  Add8 : Sum  Inputs=+++
  Add9 : Sum
  Cos : Trigonometry  Operator=cos
  Cos1 : Trigonometry  Operator=cos
  Cos2 : Trigonometry
  Cos3 : Trigonometry
  Divide : Product  Inputs=*/
  Divide1 : Product  Inputs=*/
  Exp : Math
  Gain : Gain  Gain=2
  Gain1 : Gain  Gain=2
  Gain2 : Gain  Gain=2*pi
  Gain3 : Gain  Gain=-k_a
  Max{,1,4..5} (4 alike) : MinMax  Function=max  Inputs=2
  Product{,2,7..8,11..12} (6 alike) : Product  Inputs=3
  Product{1,3..6,9..10,13..14} (9 alike) : Product
  Sqrt{,1..3} (4 alike) : Sqrt
  Square : Math  Operator=square
  Square1 : Math  Operator=square
  Square2 : Math  Operator=square
  Sum : Sum  Inputs=|+-
  下界限幅{1..2,5..6} (4 alike) : Constant  Value=1e-12
  下界限幅3 : Constant  Value=I_gate
  中心电压 : Constant  Value=V_center
  反向散射固有相移 : Constant  Value=epsilon
  激光(1)介质增益系数 : Constant  Value=alpha1
  激光(1)反向散射系数 : Constant  Value=r1
  激光(1)基准频率 : Constant  Value=sigma1
  激光(1)强度迭代-W : Integrator  InitialCondition=1
  激光(1)自饱和系数 : Constant  Value=beta1
  激光(1/2)互聚焦系数 : Constant  Value=tau12
  激光(1/2)交叉饱和系数 : Constant  Value=theta12
  激光(2)介质增益系数 : Constant  Value=alpha2
  激光(2)反向散射系数 : Constant  Value=r2
  激光(2)基准频率 : Constant  Value=sigma2
  激光(2)强度迭代 : Integrator  InitialCondition=1
  激光(2)自饱和系数 : Constant  Value=beta2
  激光(2/1)互聚焦系数 : Constant  Value=tau21
  激光(2/1)交叉饱和系数 : Constant  Value=theta21
  激光熄灭 : RelationalOperator  Operator=>  OutDataTypeStr=boolean  InputSameDT=off
  相位差迭代 : Integrator
  相位差变化率 : Outport
  光强 : Outport  Port=2
  wires:
  激光(1)介质增益系数/1 -> Product/3
  激光(1)自饱和系数/1 -> Product1/2
  Square/1 -> Product1/1
  激光(2)介质增益系数/1 -> Product2/3
  激光(2)自饱和系数/1 -> Product3/2
  Square1/1 -> Product3/1
  激光(1/2)交叉饱和系数/1 -> Product5/2
  激光(2/1)交叉饱和系数/1 -> Product6/2
  下界限幅1/1 -> Max/1
  Product4/1 -> Product6/1, Sqrt1/1, Product5/1, Sqrt/1
  激光(2)反向散射系数/1 -> Gain/1, Product11/1
  Gain/1 -> Product7/2
  Max5/1 -> Product7/1
  Cos/1 -> Product7/3
  Add/1 -> Cos/1
  反向散射固有相移/1 -> Add1/2, Add6/1, Add5/1, Add/2
  Cos1/1 -> Product8/3
  Max4/1 -> Product8/1
  Add1/1 -> Cos1/1
  Gain1/1 -> Product8/2
  激光(1)反向散射系数/1 -> Product12/3, Gain1/1
  下界限幅2/1 -> Max1/1
  Product/1 -> Add2/1
  Product1/1 -> Add2/2
  Product5/1 -> Add2/3
  Add2/1 -> 激光(1)强度迭代-W/1
  Product2/1 -> Add3/1
  Product3/1 -> Add3/2
  Product6/1 -> Add3/3
  Product8/1 -> Add3/4
  Add3/1 -> 激光(2)强度迭代/1
  激光(2/1)互聚焦系数/1 -> Product9/2
  激光(1/2)互聚焦系数/1 -> Product10/2
  Product7/1 -> Add2/4
  Add5/1 -> Cos2/1
  Max/1 -> Add9/1, Product9/1, Divide1/2, Divide/1, Product/2, Square/1, Product4/1
  Divide/1 -> Sqrt2/1
  Cos2/1 -> Product11/2
  相位差迭代/1 -> Add1/1, Add6/2, Add5/2, Add/1
  Add6/1 -> Cos3/1
  Divide1/1 -> Sqrt3/1
  Cos3/1 -> Product12/2
  激光(1)基准频率/1 -> Add4/2
  激光(2)基准频率/1 -> Add4/3
  Product14/1 -> Add4/1
  Product9/1 -> Add7/1
  Product10/1 -> Add7/5
  Product11/1 -> Add7/2
  Product12/1 -> Add7/4
  Add4/1 -> Add7/3
  Add7/1 -> 相位差变化率/1, 相位差迭代/1
  激光(1)强度迭代-W/1 -> Max/2
  激光(2)强度迭代/1 -> Max1/2
  下界限幅5/1 -> Max4/1
  Sqrt1/1 -> Max4/2
  下界限幅6/1 -> Max5/1
  Sqrt/1 -> Max5/2
  Sqrt2/1 -> Product11/3
  Sqrt3/1 -> Product12/1
  零偏速率/1 -> Add8/3
  温度标度因数/1 -> Product13/2
  本体角速度/1 -> Add8/1
  抖动角速度/1 -> Add8/2
  Add8/1 -> Gain2/1
  Gain2/1 -> Product13/1
  Max1/1 -> Product4/2, Square1/1, Product2/2, Divide/2, Divide1/1, Add9/2, Product10/1
  Add9/1 -> 光强/1, 激光熄灭/1
  Product13/1 -> Product14/2
  激光熄灭/1 -> Product14/1
  下界限幅3/1 -> 激光熄灭/2
  扫模电压/1 -> Sum/1
  中心电压/1 -> Sum/2
  Sum/1 -> Square2/1
  Gain3/1 -> Exp/1
  Exp/1 -> Product2/1, Product/1
  Square2/1 -> Gain3/1

== system satellite2/姿态确定与控制系统/三轴姿态动力学子系统/rlg_r/几何参数 ==
  Mux : Mux  Inputs=3
  激光波长-m : Constant  Value=wavelength_m
  环形腔周长-m : Constant  Value=perimeter_m
  环形腔面积-m2 : Constant  Value=area_m2
  计算集合标度因数-S0 : Fcn  Expr=4*u(1)/(u(2)*u(3))
  标度因数 : Outport
  wires:
  计算集合标度因数-S0/1 -> 标度因数/1
  Mux/1 -> 计算集合标度因数-S0/1
  环形腔面积-m2/1 -> Mux/1
  激光波长-m/1 -> Mux/2
  环形腔周长-m/1 -> Mux/3

== system satellite2/姿态确定与控制系统/三轴姿态动力学子系统/rlg_r/噪声模型 ==
  标度因数 : Inport
  相位差变化率 : Inport  Port=2
  Add : Sum
  Band-Limited White Noise : simulink/Sources/Band-Limited White Noise  Cov=[(ARW_deg_per_sqrt_h/60)^2 + white_rate_std_deg_s^2]  Ts=1  seed=[23341]
  Divide : Product  Inputs=/*
  Gain : Gain  Gain=pi/180
  r2Hz : Gain  Gain=1/(2*pi)
  测量角速度 : Outport
  wires:
  Add/1 -> 测量角速度/1
  r2Hz/1 -> Divide/2
  Gain/1 -> Add/1
  Band-Limited White Noise/1 -> Gain/1
  Divide/1 -> Add/2
  相位差变化率/1 -> r2Hz/1
  标度因数/1 -> Divide/1

== system satellite2/姿态确定与控制系统/三轴姿态动力学子系统/rlg_r/控模与扫模逻辑 ==
  光强 : Inport
  Add : Sum  Inputs=+-
  Add1 : Sum
  Gain : Gain  Gain=kP
  Gain1 : Gain  Gain=kI
  Integrator : Integrator
  Switch : Switch  Criteria=u2 > Threshold  SaturateOnIntegerOverflow=off  InputSameDT=off
  zero : Constant  Value=0  OutDataTypeStr=boolean
  光强阈值 : Constant  Value=I_triggle
  扫模信号发生器 : simulink/Sources/Repeating Sequence  rep_seq_t=[0 0.5 1]  rep_seq_y=[0 V_pzt_max V_pzt_min]
  期望光强 : Constant  Value=I_e
  状态切换 : simulink_extras/Flip Flops/S-R Flip-Flop  initial_condition=0
  触发信号 : RelationalOperator  OutDataTypeStr=boolean  RndMeth=Simplest  InputSameDT=off
  触发信号1 : RelationalOperator  Operator=<  OutDataTypeStr=boolean  RndMeth=Simplest  InputSameDT=off
  跌落阈值 : Constant  Value=I_gate
  扫模电压 : Outport
  wires:
  光强阈值/1 -> 触发信号/2
  期望光强/1 -> Add/1
  Add1/1 -> Switch/1
  状态切换/1 -> Switch/2
  扫模信号发生器/1 -> Switch/3
  触发信号/1 -> 状态切换/1
  Switch/1 -> 扫模电压/1
  Add/1 -> Gain1/1, Gain/1
  Gain/1 -> Add1/2
  Gain1/1 -> Integrator/1
  Integrator/1 -> Add1/1
  触发信号1/1 -> 状态切换/2
  光强/1 -> 触发信号1/1, Add/2, 触发信号/1
  跌落阈值/1 -> 触发信号1/2

== system satellite2/姿态确定与控制系统/三轴姿态动力学子系统/rlg_r/机械抖动 ==
  Add : Sum
  Add1 : Sum  Inputs=-+-
  Clock : Clock
  Product{,1..3,5} (5 alike) : Product
  Product6 : Product  Inputs=3
  Scope : Scope
      settings: DataLoggingVariableName=ScopeData4
  Scope1 : Scope
      settings: DataLoggingVariableName=ScopeData5
  Sin : Trigonometry
  Square : Math  Operator=square
  deg2rad : Gain  Gain=pi/180
  dither_d : ToWorkspace  VariableName=dither_d  SampleTime=-1
  dither_w : ToWorkspace  VariableName=dither_w  SampleTime=-1
  r2rad : Gain  Gain=2*pi
  倍数 : Constant  Value=2.0
  初相位 : Constant  Value=initial_phase
  抖动固有频率-Hz : Constant  Value=f_n_hz
  抖动角度迭代 : Integrator
  抖动角速度迭代 : Integrator
  抖动角速度（峰值）-deg/s : Constant  Value=v_peak_deg_s
  阻尼比 : Constant  Value=zeta
  抖动角速度 : Outport
  wires:
  r2rad/1 -> Square/1, Product6/1, Product1/2  "抖动固有角频率-rad/s"
  抖动固有频率-Hz/1 -> r2rad/1
  阻尼比/1 -> Product/2
  倍数/1 -> Product/1
  Clock/1 -> Product1/1
  Product1/1 -> Add/1
  初相位/1 -> Add/2
  Add/1 -> Sin/1
  Product3/1 -> Product2/1  "驱动力矩幅值-N·m"
  Sin/1 -> Product2/2
  Product2/1 -> Add1/2  "驱动力矩-N·m"
  deg2rad/1 -> Product3/1  "抖动角度幅值-rad"
  抖动角速度（峰值）-deg/s/1 -> deg2rad/1
  Product/1 -> Product6/2, Product3/2
  Add1/1 -> 抖动角速度迭代/1
  Product6/1 -> Add1/3
  Square/1 -> Product5/2
  抖动角度迭代/1 -> dither_d/1, Scope1/1, Product5/1
  Product5/1 -> Add1/1
  抖动角速度迭代/1 -> Scope/1, dither_w/1, Product6/3, 抖动角速度/1, 抖动角度迭代/1

== system satellite2/姿态确定与控制系统/三轴姿态动力学子系统/rlg_r/热模型 ==
  环境温度-°C : Inport
  几何标度因数 : Inport  Port=2
  Add : Sum
  Add1 : Sum  Inputs=+++
  Add2 : Sum
  Product : Product
  Sum : Sum  Inputs=|-+
  deg2rad(s) : Gain  Gain=pi/(180*3600)
  平方 : Math  Operator=square
  标定/初始温度 : Constant  Value=25
  标度因数倍数（参考温度） : Constant
  比较 : Sum  Inputs=-+|
  温度标度因数系数（1阶） : Gain  Gain=k_sf1_ppm
  温度标度因数系数（2阶） : Gain  Gain=k_sf2_ppm
  温度迭代 : Integrator  InitialConditionSource=external  InitialCondition=25.0
  温度零偏系数（1阶） : Gain  Gain=k_bias1_deg_h_per_C
  温度零偏系数（2阶） : Gain  Gain=k_bias2_deg_h_per_C
  热时间常数 : Gain  Gain=1/tau_th_s
  百万分之一每摄氏度 : Gain  Gain=1e-6
  零偏（参考温度） : Constant  Value=bias0_deg_h
  陀螺温度-°C : Outport
  温度标度因数 : Outport  Port=2
  温度零偏 : Outport  Port=3
  wires:
  热时间常数/1 -> 温度迭代/1
  温度迭代/1 -> 陀螺温度-°C/1, Sum/2, 比较/1
  环境温度-°C/1 -> 比较/2
  比较/1 -> 热时间常数/1
  温度标度因数系数（1阶）/1 -> Add/1
  温度标度因数系数（2阶）/1 -> Add/2
  标定/初始温度/1 -> Sum/1, 温度迭代/2
  Add/1 -> 百万分之一每摄氏度/1
  Product/1 -> 温度标度因数/1
  平方/1 -> 温度标度因数系数（2阶）/1, 温度零偏系数（2阶）/1
  deg2rad(s)/1 -> 温度零偏/1
  几何标度因数/1 -> Product/1
  Add1/1 -> deg2rad(s)/1
  Sum/1 -> 平方/1, 温度标度因数系数（1阶）/1, 温度零偏系数（1阶）/1
  温度零偏系数（2阶）/1 -> Add1/3
  温度零偏系数（1阶）/1 -> Add1/2
  零偏（参考温度）/1 -> Add1/1
  百万分之一每摄氏度/1 -> Add2/2
  标度因数倍数（参考温度）/1 -> Add2/1
  Add2/1 -> Product/2

== system satellite2/姿态确定与控制系统/三轴姿态动力学子系统/四元数传播-欧拉法/向量模长-q ==
  u0 : Inport
  u1 : Inport  Port=2
  u2 : Inport  Port=3
  u3 : Inport  Port=4
  Add : Sum  Inputs=4
  Sqrt : Sqrt
  Square{,1..3} (4 alike) : Math  Operator=square
  |u| : Outport
  wires:
  u0/1 -> Square/1
  u1/1 -> Square1/1
  u2/1 -> Square2/1
  Square/1 -> Add/1
  Square1/1 -> Add/2
  Square2/1 -> Add/3
  Add/1 -> Sqrt/1
  Sqrt/1 -> |u|/1
  u3/1 -> Square3/1
  Square3/1 -> Add/4

== system satellite2/姿态确定与控制系统/三轴姿态动力学子系统/四元数传播-闭式积分/四元数乘法 ==
  Q1 : Inport
  Q2 : Inport  Port=2
  Add : Sum  Inputs=3
  Cross Product : matrix_library/Cross Product
  Demux : Demux
  Demux1 : Demux
  Dot Product : DotProduct  OutDataTypeStr=Inherit: Inherit via internal rule
  Mux : Mux  Inputs=2
  Mux1 : Mux  Inputs=3
  Mux2 : Mux  Inputs=3
  Product : Product
  Product1 : Product
  Product2 : Product
  Sum : Sum  Inputs=|+-
  Q* : Outport
  wires:
  Q1/1 -> Demux/1
  Q2/1 -> Demux1/1
  Mux/1 -> Q*/1
  Product/1 -> Sum/1
  Demux/1 -> Product1/1, Product/1
  Mux1/1 -> Dot Product/1, Cross Product/1, Product2/2
  Demux1/1 -> Product2/1, Product/2
  Mux2/1 -> Cross Product/2, Dot Product/2, Product1/2
  Sum/1 -> Mux/1
  Dot Product/1 -> Sum/2
  Product2/1 -> Add/2
  Product1/1 -> Add/1
  Cross Product/1 -> Add/3
  Add/1 -> Mux/2
  Demux/2 -> Mux1/1
  Demux/3 -> Mux1/2
  Demux/4 -> Mux1/3
  Demux1/2 -> Mux2/1
  Demux1/3 -> Mux2/2
  Demux1/4 -> Mux2/3

== system satellite2/姿态确定与控制系统/重力梯度力矩/hat-r_b/向量模长-r_i ==
  u0 : Inport
  u1 : Inport  Port=2
  u2 : Inport  Port=3
  Add : Sum  Inputs=3
  Sqrt : Sqrt
  Square : Math  Operator=square
  Square1 : Math  Operator=square
  Square2 : Math  Operator=square
  |u| : Outport
  wires:
  u0/1 -> Square/1
  u1/1 -> Square1/1
  u2/1 -> Square2/1
  Square/1 -> Add/1
  Square1/1 -> Add/2
  Square2/1 -> Add/3
  Add/1 -> Sqrt/1
  Sqrt/1 -> |u|/1

== system satellite2/电源子系统/太阳能板/太阳板/伏电特性 ==
  note: $I=(N_p\cdot I_{ph})-(N_p\cdot I_0)\left(e^{\frac{V+I(N_s\cdot R_s / N_p)}{(N_s\cdot n)V_t}}-1\right)-\frac{V+I(N_s\cdot R_s / N_p)}{N_s\cdot R_{sh} / N_p}$
  lr : Inport
  V : Inport  Port=2
  Controlled Voltage Source : fl_lib/Electrical/Electrical Sources/Controlled Voltage Source
  ERef : fl_lib/Electrical/Electrical Elements/Electrical Reference
  Sensing Current : Subsystem
      mask Display: disp('i')
  Simulink-PS Converter : nesl_utility/Simulink-PS Converter  PhysicalDomain=network_engine_domain  SubClassName=ps_input  LeftPortType=input  RightPortType=output  PseudoPeriodic=off  Frequencies=[]  NoiseDistribution=none  NoiseParameters=[]  Unit=W/m^2  AffineConversion=off  FilteringAndDerivatives=provide  SimscapeFilterOrder=1  InputFilterTimeConstant=0.01  UdotUserProvided=0
  Simulink-PS Converter1 : nesl_utility/Simulink-PS Converter  PhysicalDomain=network_engine_domain  SubClassName=ps_input  LeftPortType=input  RightPortType=output  PseudoPeriodic=off  Frequencies=[]  NoiseDistribution=none  NoiseParameters=[]  Unit=1  AffineConversion=off  FilteringAndDerivatives=zero  SimscapeFilterOrder=1  InputFilterTimeConstant=0.001  UdotUserProvided=1
  Solar Cell1 : ee_lib/Sources/Solar Cell  prm=ee.enum.sources.solar_cell_prm.eightParameter  Isc=3.8 A  Voc=0.586 V  Is=I_f A  Is2=0 A  Iph=I_sc A  Ir0=G0 W/m^2  ec=n  N2=2  Rs=R_s Ohm  Rp=R_p Ohm  N_series=num_s  N_parallel=num_p  TIPH1=0.000805 1/K  EG=1.14 eV  TXIS1=3.38  TXIS2=3  TRS1=0  TRP1=0  Tmeas=25 degC  TFIXED=25 degC  thermal_mass=100 J/K  initial_temperature=25 degC
  Solver Configuration : nesl_utility/Solver Configuration  PhysicalDomain=network_engine_domain  SubClassName=solver  LeftPortType=input  RightPortType=generic  Tones=[]  Harmonics=[]  SimulateNoise=off  Profile=off  UseLocalSampling=off  EnableSwitchedLinearOptims=on  FrequencyDomain=off  UseCCode=off  RelTol=0.001  AbsTol=1e-06  MinStep=1e-09  ToWorkspace=off  RevertToSquareIcSolve=off  NumHomotopyIterations=100  PhasorMode=off  PhasorModeNumHarmonics=1  ConsistencySolver=NEWTON_FTOL  IndexReductionMethod=DerivativeReplacement  DoDC=off  ResidualTolerance=1e-9  ConsistencyTolSource=GLOBAL  ConsistencyAbsTol=0.001  ConsistencyRelTol=0.001  ConsistencyTolFactor=0.001  UseLocalSolver=off  LocalSolverChoice=NE_BACKWARD_EULER_ADVANCER  ResolveIndetEquations=on  FunctionEvalNumThread=1  LocalSolverSampleTime=0.1  DoFixedCost=off  MaxNonlinIter=3  MaxModeIter=2  ComputeImpulses=off  ImpulseIterations=2  LinearAlgebra=auto  LinearAlgebraNumThread=0  EquationFormulation=NE_TIME_EF  DelaysMemoryBudget=1024  AutomaticFiltering=on  FilteringTimeConstant=0.001  PartitionStorageMethod=AS_NEEDED  PartitionMemoryBudget=1024  PartitionMethod=FAST  MultibodyUseLocalSolver=off  MultibodyLocalSolverChoice=ODE1  MultibodyLocalSolverSampleTime=0.001
  I : Outport
  wires:
  lr/1 -> Simulink-PS Converter/1
  Sensing Current/1(Out1) -> I/1
  V/1 -> Simulink-PS Converter1/1
  connections:
  Simulink-PS Converter/RConn1 -- Solar Cell1/LConn1
  Sensing Current/LConn1 -- Solar Cell1/LConn2
  Simulink-PS Converter1/RConn1 -- Controlled Voltage Source/RConn1
  Controlled Voltage Source/LConn1 -- Sensing Current/RConn1
  Controlled Voltage Source/RConn2 -- ERef/LConn1 -- Solar Cell1/RConn1 -- Solver Configuration/RConn1

== system satellite2/电源子系统/太阳能板/太阳板/入射角余弦 ==
  note: $\hat{s}_b=q^*\otimes\hat{s}_i\otimes q$ 取矢量部分
  q : Inport
  Max : MinMax  Function=max  Inputs=2
  余弦夹角 : Subsystem
  共轭 : Subsystem
  四元数乘法 : Subsystem
  四元数旋转 : Subsystem
  地日矢量 : Constant  Value=[0;hat_s]
  面板法向量 : Constant  Value=n_solar
  入射角余弦 : Outport
  wires:
  四元数旋转/1(Q*) -> 余弦夹角/2(u2)
  余弦夹角/1(cos(γ)) -> Max/1
  四元数乘法/1(Q*) -> 四元数旋转/1(Q1)
  q/1 -> 四元数旋转/2(Q2), 共轭/1(q)
  面板法向量/1 -> 余弦夹角/1(u1)
  共轭/1(q*) -> 四元数乘法/1(Q1)
  地日矢量/1 -> 四元数乘法/2(Q2)
  Max/1 -> 入射角余弦/1
  [zero] -> Max/2

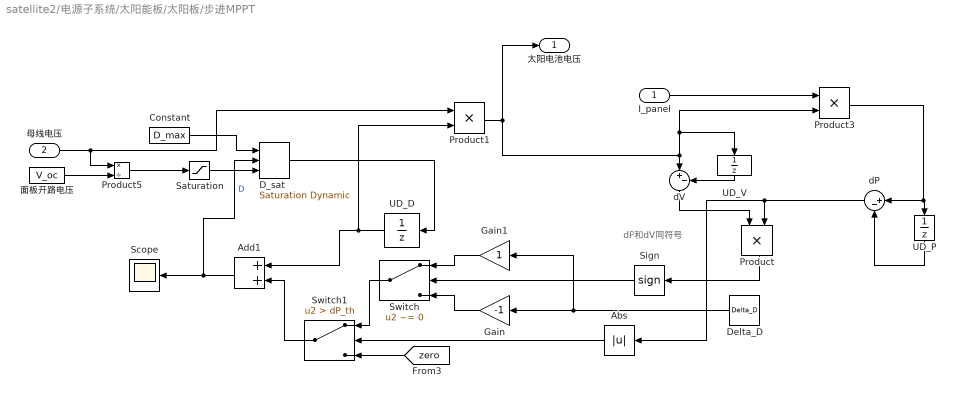
== system satellite2/电源子系统/太阳能板/太阳板/步进MPPT ==
  note: dP和dV同符号
  I_panel : Inport
  母线电压 : Inport  Port=2
  Abs : Abs  SaturateOnIntegerOverflow=off
  Add1 : Sum
  Constant : Constant  Value=D_max
  D_sat : simulink/Discontinuities/Saturation Dynamic  OutMin=[]  OutMax=[D_max]  OutDataTypeStr=Inherit: Same as second input  OutDataType=fixdt(1, 16)  OutScaling=2^-10  DoSatur=off
  Delta_D : Constant  Value=Delta_D
  Gain : Gain  Gain=-1
  Gain1 : Gain
  Product : Product
  Product1 : Product
  Product3 : Product
  Product5 : Product  Inputs=*/
  Saturation : Saturate  UpperLimit=1  LowerLimit=0
  Scope : Scope
      settings: ActiveDisplayYMinimum=0.43850000000000011  ActiveDisplayYMaximum=1.0635  DataLoggingVariableName=ScopeData7
  Sign : Signum
  Switch : Switch  Criteria=u2 ~= 0  SaturateOnIntegerOverflow=off  InputSameDT=off
  Switch1 : Switch  Criteria=u2 > Threshold  Threshold=dP_th  SaturateOnIntegerOverflow=off  InputSameDT=off
  UD_D : UnitDelay  InitialCondition=0.5  SampleTime=-1  HasFrameUpgradeWarning=on
  UD_P : UnitDelay  SampleTime=-1  HasFrameUpgradeWarning=on
  UD_V : UnitDelay  SampleTime=-1  HasFrameUpgradeWarning=on
  dP : Sum  Inputs=|+-
  dV : Sum  Inputs=|+-
  面板开路电压 : Constant  Value=V_oc
  太阳电池电压 : Outport
  wires:
  Product5/1 -> Saturation/1
  UD_D/1 -> Product1/2, Add1/1
  Switch/1 -> Switch1/1
  Product3/1 -> dP/1, UD_P/1
  Product1/1 -> 太阳电池电压/1, Product3/2, UD_V/1, dV/1
  Add1/1 -> D_sat/2, Scope/1  "D"
  dV/1 -> Product/1
  UD_V/1 -> dV/2
  UD_P/1 -> dP/2
  Gain1/1 -> Switch/1
  Abs/1 -> Switch1/2
  Saturation/1 -> D_sat/3
  Constant/1 -> D_sat/1
  dP/1 -> Abs/1, Product/2
  Delta_D/1 -> Gain1/1, Gain/1
  Product/1 -> Sign/1
  母线电压/1 -> Product1/1, Product5/1
  D_sat/1 -> UD_D/1
  面板开路电压/1 -> Product5/2
  Gain/1 -> Switch/3
  [zero] -> Switch1/3
  Switch1/1 -> Add1/2
  Sign/1 -> Switch/2
  I_panel/1 -> Product3/1

== system satellite2/电源子系统/视线角标志/余弦夹角/向量模长-r1 ==
  u1 : Inport
  u2 : Inport  Port=2
  u3 : Inport  Port=3
  Add : Sum  Inputs=+++
  Sqrt : Sqrt
  Square : Math  Operator=square
  Square1 : Math  Operator=square
  Square2 : Math  Operator=square
  |u| : Outport
  wires:
  Sqrt/1 -> |u|/1
  Add/1 -> Sqrt/1
  Square2/1 -> Add/3
  Square1/1 -> Add/2
  Square/1 -> Add/1
  u3/1 -> Square2/1
  u2/1 -> Square1/1
  u1/1 -> Square/1

== system satellite2/电源子系统/视线角标志/余弦夹角/向量模长-r2 ==
  u1 : Inport
  u2 : Inport  Port=2
  u3 : Inport  Port=3
  Add : Sum  Inputs=+++
  Sqrt : Sqrt
  Square : Math  Operator=square
  Square1 : Math  Operator=square
  Square2 : Math  Operator=square
  |u| : Outport
  wires:
  u1/1 -> Square/1
  u2/1 -> Square1/1
  u3/1 -> Square2/1
  Square/1 -> Add/1
  Square1/1 -> Add/2
  Square2/1 -> Add/3
  Add/1 -> Sqrt/1
  Sqrt/1 -> |u|/1

== system satellite2/电源子系统/太阳能板/太阳板/伏电特性/Sensing Current ==
  Current Sensor : fl_lib/Electrical/Electrical Sensors/Current Sensor
  PS-Simulink/I : nesl_utility/PS-Simulink Converter  PhysicalDomain=network_engine_domain  SubClassName=ps_output  LeftPortType=input  RightPortType=output  PseudoPeriodic=off  Frequencies=[]  VectorFormat=1-D array  Unit=1  AffineConversion=off
  Conn1 : PMIOPort  Side=Left
  Conn2 : PMIOPort  Port=2  Side=Right
  Out1 : Outport  VectorParamsAs1DForOutWhenUnconnected=off
  wires:
  PS-Simulink/I/1 -> Out1/1
  connections:
  Current Sensor/RConn1 -- PS-Simulink/I/LConn1
  Current Sensor/LConn1 -- Conn1/RConn1
  Conn2/RConn1 -- Current Sensor/RConn2

== system satellite2/电源子系统/太阳能板/太阳板/入射角余弦/余弦夹角 ==
  u1 : Inport
  u2 : Inport  Port=2
  Demux : Demux  Outputs=3
  Demux1 : Demux  Outputs=3
  Dot Product : DotProduct  OutDataTypeStr=Inherit: Inherit via internal rule
  余弦夹角 : Product  Inputs=/*/
  向量模长-r1 : Subsystem
  向量模长-r2 : Subsystem
  cos(γ) : Outport
  wires:
  向量模长-r2/1(|u|) -> 余弦夹角/3
  Demux/3 -> 向量模长-r1/3(u3)
  Demux/2 -> 向量模长-r1/2(u2)
  Dot Product/1 -> 余弦夹角/2
  Demux/1 -> 向量模长-r1/1(u1)
  向量模长-r1/1(|u|) -> 余弦夹角/1
  u2/1 -> Dot Product/2, Demux1/1
  Demux1/1 -> 向量模长-r2/1(u1)
  Demux1/2 -> 向量模长-r2/2(u2)
  Demux1/3 -> 向量模长-r2/3(u3)
  u1/1 -> Dot Product/1, Demux/1
  余弦夹角/1 -> cos(γ)/1

== system satellite2/电源子系统/太阳能板/太阳板/入射角余弦/共轭 ==
  q : Inport
  -qd1 : Gain  Gain=-1
  -qd2 : Gain  Gain=-1
  -qd3 : Gain  Gain=-1
  Demux : Demux
  Mux : Mux
  q* : Outport
  wires:
  q/1 -> Demux/1
  Mux/1 -> q*/1
  Demux/1 -> Mux/1
  Demux/2 -> -qd1/1
  -qd1/1 -> Mux/2
  Demux/3 -> -qd2/1
  -qd2/1 -> Mux/3
  Demux/4 -> -qd3/1
  -qd3/1 -> Mux/4

== system satellite2/电源子系统/太阳能板/太阳板/入射角余弦/四元数乘法 ==
  Q1 : Inport
  Q2 : Inport  Port=2
  Add : Sum  Inputs=3
  Cross Product : matrix_library/Cross Product
  Demux : Demux
  Demux1 : Demux
  Dot Product : DotProduct  OutDataTypeStr=Inherit: Inherit via internal rule
  Mux : Mux  Inputs=2
  Mux1 : Mux  Inputs=3
  Mux2 : Mux  Inputs=3
  Product : Product
  Product1 : Product
  Product2 : Product
  Sum : Sum  Inputs=|+-
  Q* : Outport
  wires:
  Q1/1 -> Demux/1
  Q2/1 -> Demux1/1
  Mux/1 -> Q*/1
  Product/1 -> Sum/1
  Demux/1 -> Product1/1, Product/1
  Mux1/1 -> Dot Product/1, Cross Product/1, Product2/2
  Demux1/1 -> Product2/1, Product/2
  Mux2/1 -> Cross Product/2, Dot Product/2, Product1/2
  Sum/1 -> Mux/1
  Dot Product/1 -> Sum/2
  Product2/1 -> Add/2
  Product1/1 -> Add/1
  Cross Product/1 -> Add/3
  Add/1 -> Mux/2
  Demux/2 -> Mux1/1
  Demux/3 -> Mux1/2
  Demux/4 -> Mux1/3
  Demux1/2 -> Mux2/1
  Demux1/3 -> Mux2/2
  Demux1/4 -> Mux2/3

== system satellite2/电源子系统/太阳能板/太阳板/入射角余弦/四元数旋转 ==
  Q1 : Inport
  Q2 : Inport  Port=2
  Add : Sum  Inputs=3
  Cross Product : matrix_library/Cross Product
  Demux : Demux
  Demux1 : Demux
  Mux1 : Mux  Inputs=3
  Mux2 : Mux  Inputs=3
  Product1 : Product
  Product2 : Product
  Q* : Outport
  wires:
  Demux1/4 -> Mux2/3
  Demux1/3 -> Mux2/2
  Demux1/2 -> Mux2/1
  Demux/4 -> Mux1/3
  Demux/3 -> Mux1/2
  Demux/2 -> Mux1/1
  Add/1 -> Q*/1
  Cross Product/1 -> Add/3
  Product1/1 -> Add/1
  Product2/1 -> Add/2
  Mux2/1 -> Product1/2, Cross Product/2
  Demux1/1 -> Product2/1
  Mux1/1 -> Product2/2, Cross Product/1
  Demux/1 -> Product1/1
  Q2/1 -> Demux1/1
  Q1/1 -> Demux/1

== system satellite2/电源子系统/太阳能板/太阳板/入射角余弦/余弦夹角/向量模长-r1 ==
  u1 : Inport
  u2 : Inport  Port=2
  u3 : Inport  Port=3
  Add : Sum  Inputs=+++
  Sqrt : Sqrt
  Square : Math  Operator=square
  Square1 : Math  Operator=square
  Square2 : Math  Operator=square
  |u| : Outport
  wires:
  Sqrt/1 -> |u|/1
  Add/1 -> Sqrt/1
  Square2/1 -> Add/3
  Square1/1 -> Add/2
  Square/1 -> Add/1
  u3/1 -> Square2/1
  u2/1 -> Square1/1
  u1/1 -> Square/1

== system satellite2/电源子系统/太阳能板/太阳板/入射角余弦/余弦夹角/向量模长-r2 ==
  u1 : Inport
  u2 : Inport  Port=2
  u3 : Inport  Port=3
  Add : Sum  Inputs=+++
  Sqrt : Sqrt
  Square : Math  Operator=square
  Square1 : Math  Operator=square
  Square2 : Math  Operator=square
  |u| : Outport
  wires:
  u1/1 -> Square/1
  u2/1 -> Square1/1
  u3/1 -> Square2/1
  Square/1 -> Add/1
  Square1/1 -> Add/2
  Square2/1 -> Add/3
  Add/1 -> Sqrt/1
  Sqrt/1 -> |u|/1
